simulink model "MPC_v02"  (R2020b)
settings: Solver=VariableStepAuto  StartTime=0.0  StopTime=24*60*60  FixedStep=60  RelTol=1e-7
values from neighbouring files (symbols this model uses):
  Atank = 1.69    [parameters.m]
  Ce = 191400    [parameters.m]
  Cp = 4180    [parameters.m]
  dx = 0.2147    [parameters.m]
  k = 469    [parameters.m]
  Kloss = 3.82    [parameters.m]
  mdot = 0.1667    [parameters.m]
  N = 5    [parameters.m]
  T0 = 40    [parameters.m]
  T_cold = 10    [parameters.m]
  UA = 0.2072    [parameters.m]
libraries: dspswit3 x1, simulink x1, mpclib x1
settings Model: Creator=enzlp  LastModifiedBy=enzlp
settings SolverCC: AlgebraicLoopSolver=LineSearch

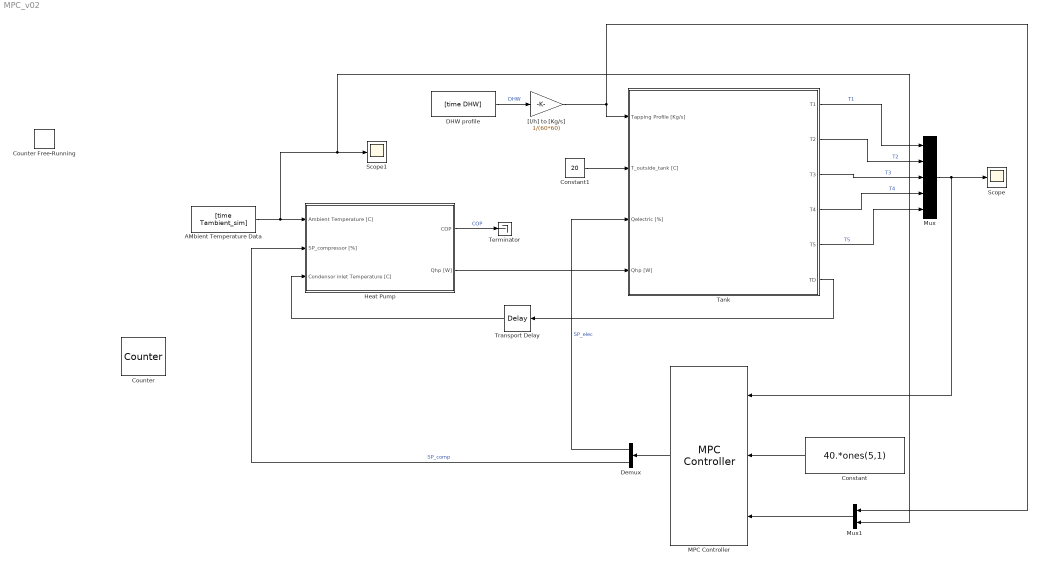
== system MPC_v02 ==
  AMbient Temperature Data : FromWorkspace  VariableName=[time Tambient_sim]  SampleTime=60
  Constant : Constant  Value=40.*ones(5,1)
  Constant1 : Constant  Value=20
  Counter : dspswit3/Counter  Direction=Up  CountEvent=Rising edge  CounterSize=User defined  MaxCount=255  InitialCount=0  Output=Count and Hit  HitValue=32  ResetInput=on  SamplesPerFrame=1  Ts=1  CntDtype=double  HitDtype=Logical
  Counter Free-Running : simulink/Sources/Counter Free-Running  NumBits=16  tsamp=-1
  DHW profile : FromWorkspace  VariableName=[time DHW]  SampleTime=60
  Demux : Demux  Outputs=2
  Heat Pump : Subsystem
  MPC Controller : mpclib/MPC Controller  SCDEnableBlockLinearizationSpecification=on  mpcobj=mpc1  is_multiple=0  enable_value=0  return_u0=off  updateMPCinCallerWorkspace=on  md_inport=on  mv_inport=off  uref_inport=off  return_cost=off  return_mvseq=off  return_qpstatus=off  return_xseq=off  return_state=off  return_ovseq=off  state_inport=off  umin_inport=off  umax_inport=off  ymin_inport=off  ymax_inport=off  cc_inport=off  ywt_inport=off  uwt_inport=off  duwt_inport=off  rhoeps_inport=off  pm_inport=off  MaximumP=10  HorizonChoice=FixedHorizon  n_ts=600  n_p=12  n_mv=2  n_md=2  n_ud=0  n_mo=5  n_uo=0  BlockDataType=double  SampleTimeInherited=off  switch_inport=off
  Mux : Mux  Inputs=5
  Mux1 : Mux  Inputs=2
  Scope : Scope
  Scope1 : Scope
  Tank : Subsystem
  Terminator : Terminator
  Transport Delay : TransportDelay  DelayTime=60  InitialOutput=40
  "[l/h] to [Kg/s]" : Gain  Gain=1/(60*60)
  wires:
  DHW profile/1 -> "[l/h] to [Kg/s]"/1  "DHW"
  Tank/3(T3) -> Mux/3  "T3"
  Tank/4(T4) -> Mux/4  "T4"
  Tank/5(T5) -> Mux/5  "T5"
  Tank/6(TD) -> Transport Delay/1
  Heat Pump/1(COP) -> Terminator/1  "COP"
  MPC Controller/1 -> Demux/1
  Demux/2 -> Heat Pump/2(SP_compressor [%])  "SP_comp"
  Demux/1 -> Tank/3(Qelectric [%])  "SP_elec"
  Tank/1(T1) -> Mux/1  "T1"
  Tank/2(T2) -> Mux/2  "T2"
  Mux/1 -> MPC Controller/1, Scope/1
  Constant/1 -> MPC Controller/2
  Constant1/1 -> Tank/2(T_outside_tank [C])
  AMbient Temperature Data/1 -> Mux1/2, Scope1/1, Heat Pump/1(Ambient Temperature [C])
  Mux1/1 -> MPC Controller/3
  "[l/h] to [Kg/s]"/1 -> Tank/1(Tapping Profile [Kg/s]), Mux1/1
  Transport Delay/1 -> Heat Pump/3(Condensor inlet Temperature [C])
  Heat Pump/2(Qhp [W]) -> Tank/4(Qhp [W])

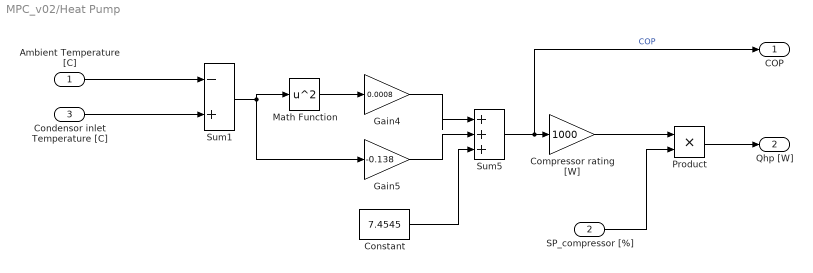
== system MPC_v02/Heat Pump ==
  Ambient Temperature [C] : Inport
  SP_compressor [%] : Inport  Port=2
  Condensor inlet Temperature [C] : Inport  Port=3
  Compressor rating [W] : Gain  Gain=1000
  Constant : Constant  Value=7.4545
  Gain4 : Gain  Gain=0.0008
  Gain5 : Gain  Gain=-0.138
  Math Function : Math  Operator=square  SignedPower=on  SaturateOnIntegerOverflow=on
  Product : Product
  Sum1 : Sum  Inputs=-+
  Sum5 : Sum  Inputs=|+++
  COP : Outport  VectorParamsAs1DForOutWhenUnconnected=off
  Qhp [W] : Outport  Port=2
  wires:
  Sum1/1 -> Math Function/1, Gain5/1
  Condensor inlet Temperature [C]/1 -> Sum1/2
  Gain4/1 -> Sum5/1
  Constant/1 -> Sum5/3
  Gain5/1 -> Sum5/2
  Sum5/1 -> Compressor rating [W]/1, COP/1  "COP"
  Ambient Temperature [C]/1 -> Sum1/1
  Math Function/1 -> Gain4/1
  Compressor rating [W]/1 -> Product/1
  Product/1 -> Qhp [W]/1
  SP_compressor [%]/1 -> Product/2

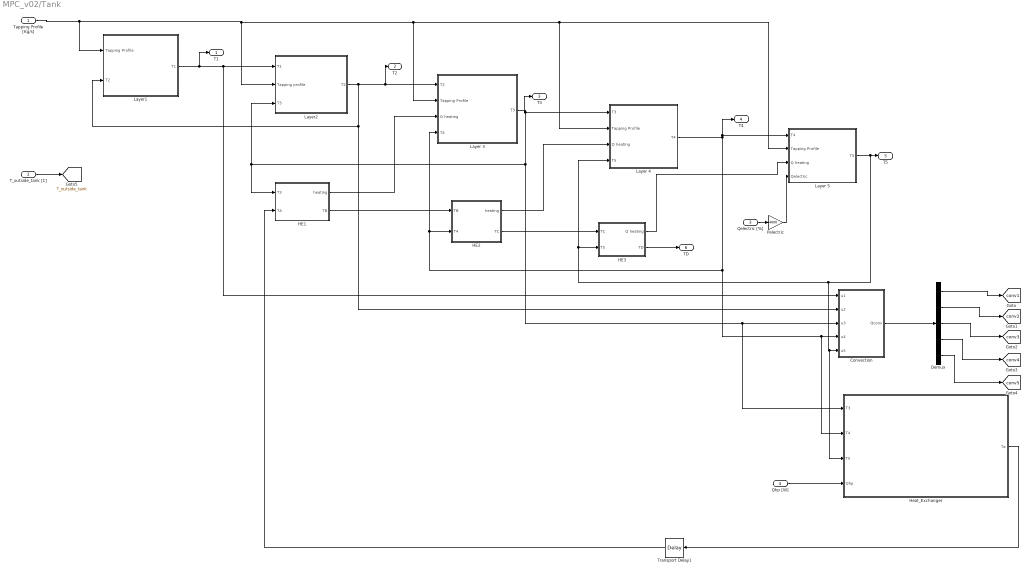
== system MPC_v02/Tank ==
  Tapping Profile [Kg/s] : Inport
  T_outside_tank [C] : Inport  Port=2
  Qelectric [%] : Inport  Port=3
  Qhp [W] : Inport  Port=4
  Convection : MATLAB Function  TreatAsAtomicUnit=on
  Demux : Demux  Outputs=5
  HE1 : Subsystem
  HE2 : Subsystem
  HE3 : Subsystem
  Heat_Exchanger : MATLAB Function  TreatAsAtomicUnit=on
  Layer 3 : Subsystem
  Layer 4 : Subsystem
  Layer 5 : Subsystem
  Layer1 : Subsystem
  Layer2 : Subsystem
  Pelectric : Gain  Gain=4000
  Transport Delay1 : TransportDelay  DelayTime=60  InitialOutput=40
  T1 : Outport
  T2 : Outport  Port=2
  T3 : Outport  Port=3
  T4 : Outport  Port=4
  T5 : Outport  Port=5
  TD : Outport  Port=6
  tag scope: T_outside_tank=global, conv1=global, conv2=global, conv3=global, conv4=global, conv5=global
  wires:
  Tapping Profile [Kg/s]/1 -> Layer 5/2(Tapping Profile), Layer 4/2(Tapping Profile), Layer 3/2(Tapping Profile), Layer2/2(Tapping profile), Layer1/1(Tapping Profile)
  HE1/2(TB) -> HE2/1(TB)
  Layer 4/1(T4) -> T4/1, Layer 5/1(T4), Layer 3/4(T4), HE2/2(T4), Heat_Exchanger/2(T4), Convection/4(u4)
  Layer1/1(T1) -> T1/1, Convection/1(u1), Layer2/1(T1)
  Layer2/1(T2) -> Convection/2(u2), Layer1/2(T2), T2/1, Layer 3/1(T2)
  Layer 5/1(T5) -> T5/1, Heat_Exchanger/3(T5), Convection/5(u5), Layer 4/4(T5), HE3/2(T5)
  Demux/2 -> [conv2]
  Demux/1 -> [conv1]
  HE2/2(TC) -> HE3/1(TC)
  Demux/5 -> [conv5]
  Demux/4 -> [conv4]
  HE3/1(Q heating) -> Layer 5/3(Q heating)
  Demux/3 -> [conv3]
  HE2/1(heating) -> Layer 4/3(Q heating)
  HE1/1(heating) -> Layer 3/3(Q heating)
  HE3/2(TD) -> TD/1
  Heat_Exchanger/1(Ta) -> Transport Delay1/1
  Convection/1(Qconv) -> Demux/1
  Qelectric [%]/1 -> Pelectric/1
  Pelectric/1 -> Layer 5/4(Qelectric)
  T_outside_tank [C]/1 -> [T_outside_tank]
  Qhp [W]/1 -> Heat_Exchanger/4(Qhp)
  Transport Delay1/1 -> HE1/2(TA)
  Layer 3/1(T3) -> Layer 4/1(T3), T3/1, HE1/1(T3), Layer2/3(T3), Heat_Exchanger/1(T3), Convection/3(u3)

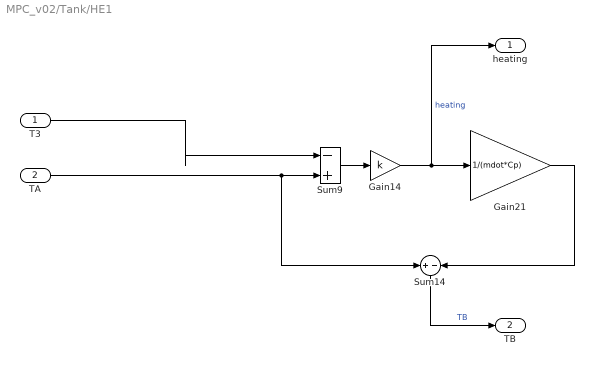
== system MPC_v02/Tank/HE1 ==
  T3 : Inport
  TA : Inport  Port=2
  Gain14 : Gain  Gain=k
  Gain21 : Gain  Gain=1/(mdot*Cp)
  Sum14 : Sum  Inputs=+|-
  Sum9 : Sum  Inputs=|-+
  heating : Outport
  TB : Outport  Port=2
  wires:
  Gain14/1 -> Gain21/1, heating/1  "heating"
  TA/1 -> Sum14/1, Sum9/2
  Sum9/1 -> Gain14/1
  Gain21/1 -> Sum14/2
  Sum14/1 -> TB/1  "TB"
  T3/1 -> Sum9/1

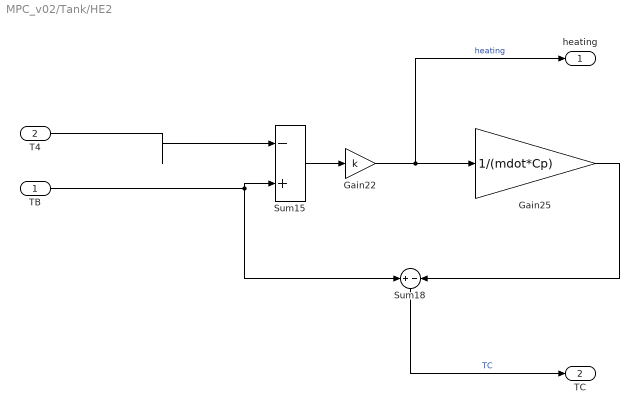
== system MPC_v02/Tank/HE2 ==
  TB : Inport
  T4 : Inport  Port=2
  Gain22 : Gain  Gain=k
  Gain25 : Gain  Gain=1/(mdot*Cp)
  Sum15 : Sum  Inputs=|-+
  Sum18 : Sum  Inputs=+|-
  heating : Outport
  TC : Outport  Port=2
  wires:
  Gain25/1 -> Sum18/2
  T4/1 -> Sum15/1
  TB/1 -> Sum15/2, Sum18/1
  Gain22/1 -> heating/1, Gain25/1  "heating"
  Sum18/1 -> TC/1  "TC"
  Sum15/1 -> Gain22/1

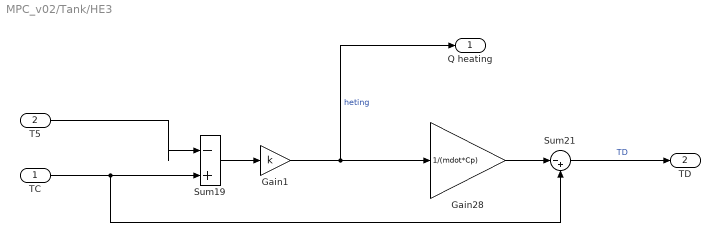
== system MPC_v02/Tank/HE3 ==
  TC : Inport
  T5 : Inport  Port=2
  Gain1 : Gain  Gain=k
  Gain28 : Gain  Gain=1/(mdot*Cp)
  Sum19 : Sum  Inputs=|-+
  Sum21 : Sum  Inputs=|-+
  Q heating : Outport
  TD : Outport  Port=2
  wires:
  TC/1 -> Sum19/2, Sum21/2
  Gain1/1 -> Gain28/1, Q heating/1  "heting"
  Gain28/1 -> Sum21/1
  T5/1 -> Sum19/1
  Sum21/1 -> TD/1  "TD"
  Sum19/1 -> Gain1/1

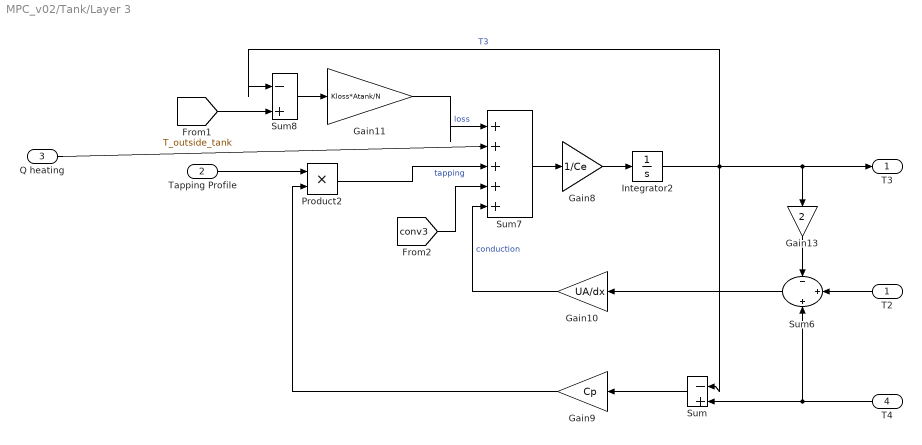
== system MPC_v02/Tank/Layer 3 ==
  T2 : Inport
  Tapping Profile : Inport  Port=2
  Q heating : Inport  Port=3
  T4 : Inport  Port=4
  Gain10 : Gain  Gain=UA/dx
  Gain11 : Gain  Gain=Kloss*Atank/N
  Gain13 : Gain  Gain=2
  Gain8 : Gain  Gain=1/Ce
  Gain9 : Gain  Gain=Cp
  Integrator2 : Integrator  InitialCondition=T0
  Product2 : Product
  Sum : Sum  Inputs=|-+
  Sum6 : Sum  Inputs=-|+|+
  Sum7 : Sum  Inputs=|+++++
  Sum8 : Sum  Inputs=|-+
  T3 : Outport
  wires:
  Product2/1 -> Sum7/3  "tapping"
  Gain11/1 -> Sum7/1  "loss"
  Gain8/1 -> Integrator2/1
  [conv3] -> Sum7/4
  Sum7/1 -> Gain8/1
  Sum6/1 -> Gain10/1
  Gain10/1 -> Sum7/5  "conduction"
  Integrator2/1 -> T3/1, Gain13/1, Sum8/1, Sum/1  "T3"
  Gain13/1 -> Sum6/1
  Q heating/1 -> Sum7/2
  Sum8/1 -> Gain11/1
  Gain9/1 -> Product2/2
  T2/1 -> Sum6/2
  Tapping Profile/1 -> Product2/1
  T4/1 -> Sum/2, Sum6/3
  Sum/1 -> Gain9/1
  [T_outside_tank] -> Sum8/2

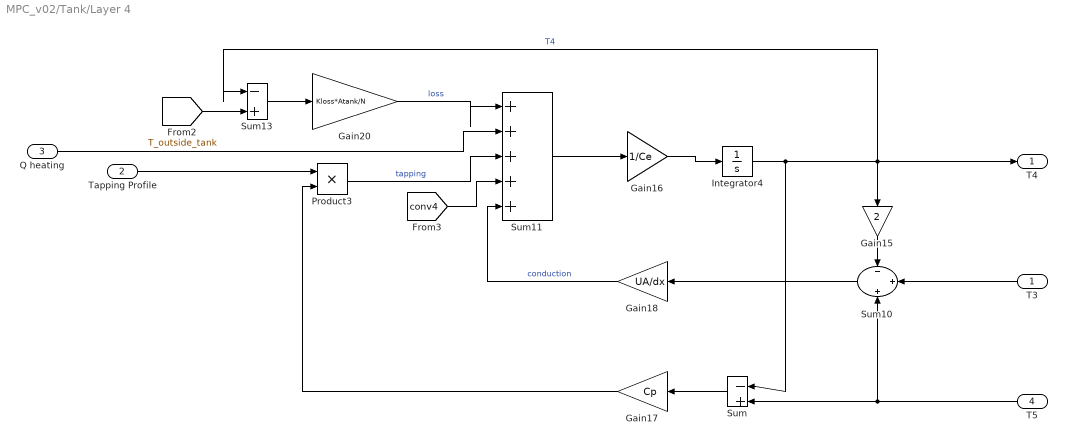
== system MPC_v02/Tank/Layer 4 ==
  T3 : Inport
  Tapping Profile : Inport  Port=2
  Q heating : Inport  Port=3
  T5 : Inport  Port=4
  Gain15 : Gain  Gain=2
  Gain16 : Gain  Gain=1/Ce
  Gain17 : Gain  Gain=Cp
  Gain18 : Gain  Gain=UA/dx
  Gain20 : Gain  Gain=Kloss*Atank/N
  Integrator4 : Integrator  InitialCondition=T0
  Product3 : Product
  Sum : Sum  Inputs=|-+
  Sum10 : Sum  Inputs=-|+|+
  Sum11 : Sum  Inputs=|+++++
  Sum13 : Sum  Inputs=|-+
  T4 : Outport
  wires:
  Gain17/1 -> Product3/2
  Gain16/1 -> Integrator4/1
  Sum10/1 -> Gain18/1
  Gain15/1 -> Sum10/1
  Sum11/1 -> Gain16/1
  Product3/1 -> Sum11/3  "tapping"
  T5/1 -> Sum/2, Sum10/3
  Gain20/1 -> Sum11/1  "loss"
  Tapping Profile/1 -> Product3/1
  Integrator4/1 -> Sum13/1, Gain15/1, T4/1, Sum/1  "T4"
  [conv4] -> Sum11/4
  Sum13/1 -> Gain20/1
  Q heating/1 -> Sum11/2
  Gain18/1 -> Sum11/5  "conduction"
  T3/1 -> Sum10/2
  Sum/1 -> Gain17/1
  [T_outside_tank] -> Sum13/2

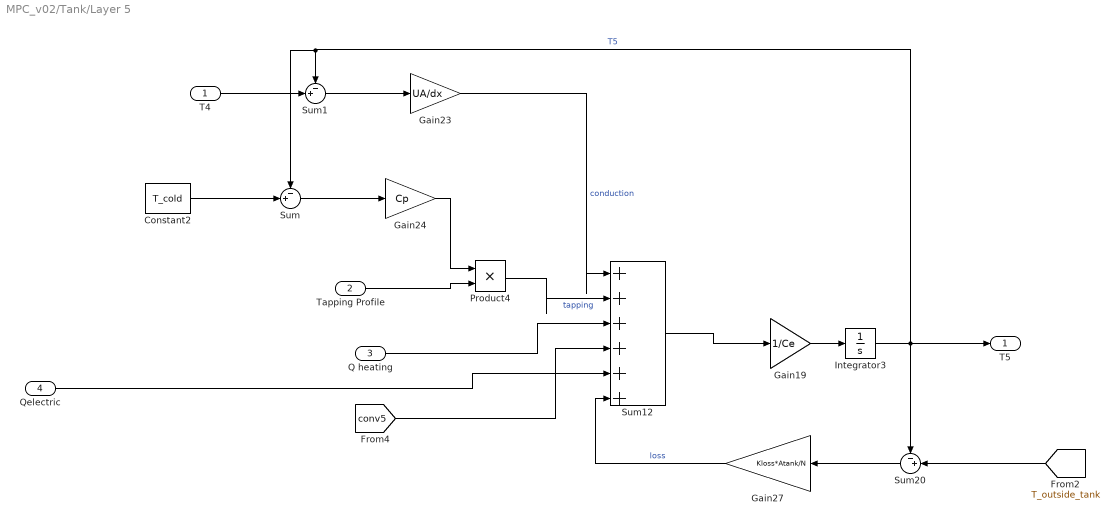
== system MPC_v02/Tank/Layer 5 ==
  T4 : Inport
  Tapping Profile : Inport  Port=2
  Q heating : Inport  Port=3
  Qelectric : Inport  Port=4
  Constant2 : Constant  Value=T_cold
  Gain19 : Gain  Gain=1/Ce
  Gain23 : Gain  Gain=UA/dx
  Gain24 : Gain  Gain=Cp
  Gain27 : Gain  Gain=Kloss*Atank/N
  Integrator3 : Integrator  InitialCondition=T0
  Product4 : Product
  Sum : Sum  Inputs=-+|
  Sum1 : Sum  Inputs=-+|
  Sum12 : Sum  Inputs=|++++++
  Sum20 : Sum  Inputs=-+|
  T5 : Outport
  wires:
  Gain23/1 -> Sum12/1  "conduction"
  Gain19/1 -> Integrator3/1
  Tapping Profile/1 -> Product4/2
  Sum12/1 -> Gain19/1
  Sum20/1 -> Gain27/1
  Gain24/1 -> Product4/1
  Gain27/1 -> Sum12/6  "loss"
  Product4/1 -> Sum12/2  "tapping"
  [conv5] -> Sum12/4
  Integrator3/1 -> Sum/1, Sum1/1, Sum20/1, T5/1  "T5"
  Q heating/1 -> Sum12/3
  Constant2/1 -> Sum/2
  Sum/1 -> Gain24/1
  T4/1 -> Sum1/2
  Sum1/1 -> Gain23/1
  Qelectric/1 -> Sum12/5
  [T_outside_tank] -> Sum20/2

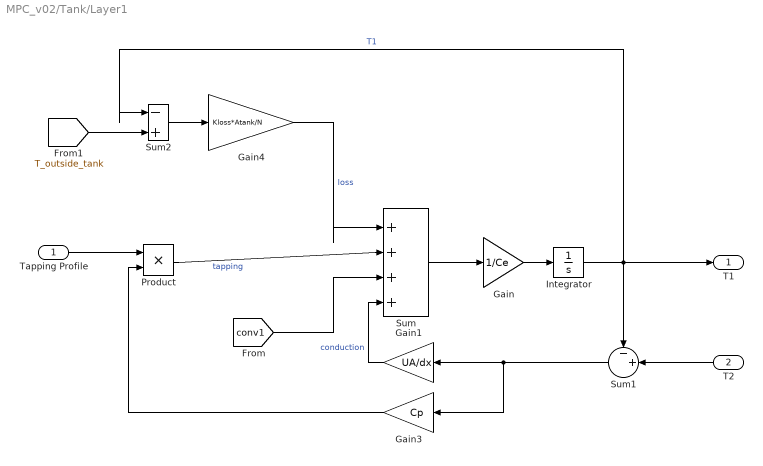
== system MPC_v02/Tank/Layer1 ==
  Tapping Profile : Inport
  T2 : Inport  Port=2
  Gain : Gain  Gain=1/Ce
  Gain1 : Gain  Gain=UA/dx
  Gain3 : Gain  Gain=Cp
  Gain4 : Gain  Gain=Kloss*Atank/N
  Integrator : Integrator  InitialCondition=T0
  Product : Product
  Sum : Sum  Inputs=|++++
  Sum1 : Sum  Inputs=-+|
  Sum2 : Sum  Inputs=|-+
  T1 : Outport
  wires:
  Sum/1 -> Gain/1
  Sum1/1 -> Gain3/1, Gain1/1
  Gain3/1 -> Product/2
  Integrator/1 -> Sum1/1, T1/1, Sum2/1  "T1"
  Gain4/1 -> Sum/1  "loss"
  Gain/1 -> Integrator/1
  Sum2/1 -> Gain4/1
  Product/1 -> Sum/2  "tapping"
  Gain1/1 -> Sum/4  "conduction"
  [conv1] -> Sum/3
  T2/1 -> Sum1/2
  Tapping Profile/1 -> Product/1
  [T_outside_tank] -> Sum2/2

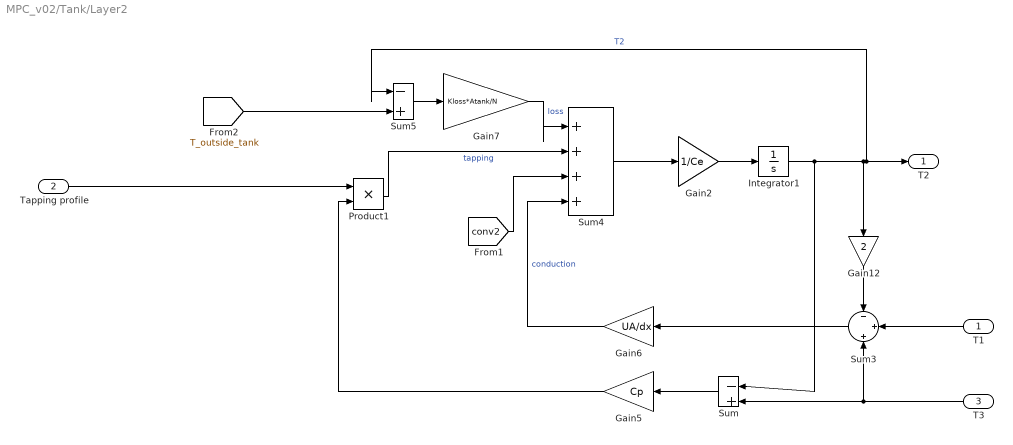
== system MPC_v02/Tank/Layer2 ==
  T1 : Inport
  Tapping profile : Inport  Port=2
  T3 : Inport  Port=3
  Gain12 : Gain  Gain=2
  Gain2 : Gain  Gain=1/Ce
  Gain5 : Gain  Gain=Cp
  Gain6 : Gain  Gain=UA/dx
  Gain7 : Gain  Gain=Kloss*Atank/N
  Integrator1 : Integrator  InitialCondition=T0
  Product1 : Product
  Sum : Sum  Inputs=|-+
  Sum3 : Sum  Inputs=-|+|+
  Sum4 : Sum  Inputs=|++++
  Sum5 : Sum  Inputs=|-+
  T2 : Outport
  wires:
  Gain12/1 -> Sum3/1
  Sum3/1 -> Gain6/1
  Gain2/1 -> Integrator1/1
  Integrator1/1 -> Sum/1, T2/1, Sum5/1, Gain12/1  "T2"
  Gain5/1 -> Product1/2
  Sum5/1 -> Gain7/1
  T1/1 -> Sum3/2
  Sum4/1 -> Gain2/1
  Gain7/1 -> Sum4/1  "loss"
  Product1/1 -> Sum4/2  "tapping"
  [conv2] -> Sum4/3
  Gain6/1 -> Sum4/4  "conduction"
  Tapping profile/1 -> Product1/1
  T3/1 -> Sum/2, Sum3/3
  Sum/1 -> Gain5/1
  [T_outside_tank] -> Sum5/2

== matlab function MPC_v02/Tank/Heat_Exchanger ==
  data: T3 input; Ta output; T4 input; T5 input; Qhp input
function Ta = fcn(T3,T4,T5,Qhp)
% Heat conduction coefficient of heating coil [W/K]
k = 469;
% Specific heat coefficient (at constant pressure) of water [J/Kg K]
Cp =4180;
% Mass flow of heating water through coil [Kg/s]
m= 0.1667;

Ta = ( (Qhp/k) + T5 - T4*(k/(m*Cp) - 1) -T3*(-1 + 2*k/(m*Cp) - k^2/(m^2*Cp^2)) ) / (3 - (3*k/(m*Cp)) + (k^2/(m^2*Cp^2)));

== matlab function MPC_v02/Tank/Convection ==
  data: u1 input; Qconv output; u2 input; u3 input; u4 input; u5 input
function Qconv = fcn(u1,u2,u3,u4,u5)

tau = 10;
C = 191400;
U = [u1 u2 u3 u4 u5];
Qconv = zeros(5,1);
index = 1;

for i=4:-1:1
    if U(i+1)>= U(i)
        index = i+1;
        break
    end
end

if i == 1            % if the loop finishes without finding inversion
    Qconv= zeros(5,1);   % no convection flux
    return 
else
    Tmean = sum(U(1:index))/index;
    for j= 5:-1:1
        if j>i
            Qconv(j)=0;
        else
            Qconv(j) = (Tmean - U(j))*C/tau;
        end
    end
end
